simulink model "Planta_FTV_load_balanceada"  (R2020a)
settings: Solver=VariableStepAuto  StartTime=0.0  StopTime=total_sim  MaxStep=1e-4  RelTol=1e-3
values from neighbouring files (symbols this model uses):
  day = 9 + i    [main.m]
  duty_solar = (4*rand())-(3*rand())+90    [main.m]
  gain_time = 0.0001    [main.m]
  L1 = 8.5e-03 + rand()*1e-04    [main.m]
  L2 = 12e-03 + rand()*1e-04    [main.m]
  L3 = 19e-03 + rand()*1e-04    [main.m]
  L4 = 18e-03 + rand()*1e-04    [main.m]
  L5 = 12e-03 + rand()*1e-04    [main.m]
  R = 10    [main.m]
  T1 = 2 *time_hour + rand()*0.5    [main.m]
  T2 = 6 *time_hour + rand()*0.5    [main.m]
  T3 = 11 *time_hour + rand()*0.5    [main.m]
  T4 = 17 * time_hour + rand()*0.5    [main.m]
  T5 = 18    [main.m]
  total_sim = (horas_simular*60*60)*gain_time    (= 0.18)    [main.m]
  ts_save = gain_time *10    (= 0.001)    [main.m]
  ts_send = 0.01    [main.m]
  weekday = 1 +i    [main.m]
libraries: powerlib x45, powerlib_meascontrol x9, simulink x2, instrumentlib x2, eePowerMeasurement x1, powerlib_extras x1, re_lib x1
settings Model: Creator=Daniel Gusnay  LastModifiedBy=bazur
settings DataIOCC: ReturnWorkspaceOutputs=off
settings DebuggingCC: ArithmeticOperatorsInVariantConditions=warning
settings SFSimCC: SimUseLocalCustomCode=off  CustomCodeUndefinedFunction=UseInterfaceOnly
settings RTWCC: RTWUseLocalCustomCode=off

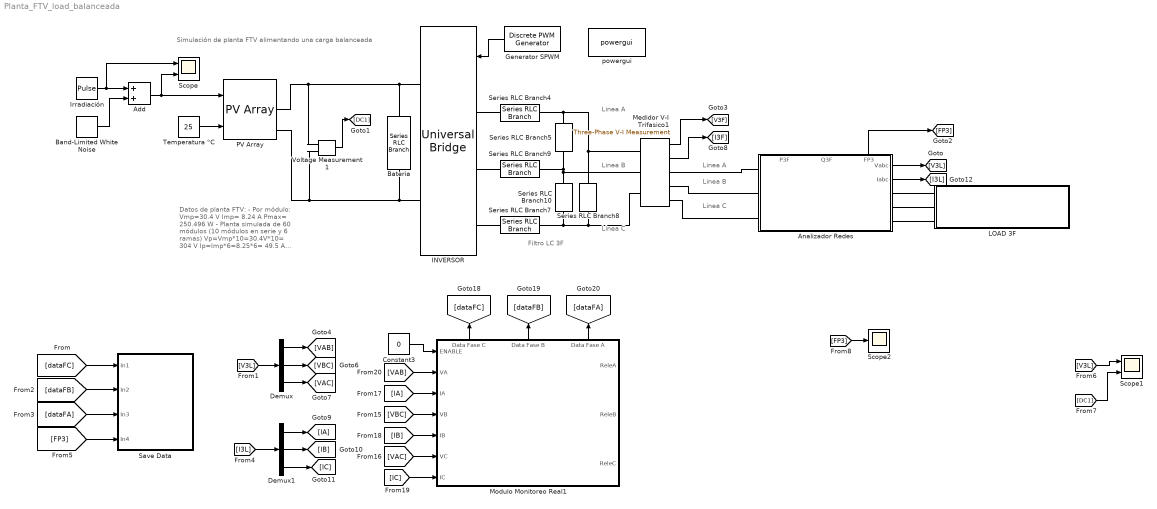
== system Planta_FTV_load_balanceada ==
  note: Simulación de planta FTV alimentando una carga balanceada
  note: Filtro LC 3F
  note: Datos de planta FTV:
      | - Por módulo:
      | Vmp=30.4 V
      | Imp= 8.24 A
      | Pmax= 250.496 W
      | - Planta simulada de 60 módulos
      | (10 módulos en serie y 6 ramas)
      | Vp=Vmp*10=30.4V*10= 304 V
      | Ip=Imp*6=8.25*6= 49.5 A
      | Pp=250.496*60= 15.03 KW
  note: Linea C
  note: Linea A
  note: Linea B
  note: Linea B
  note: Linea C
  note: Linea A
  Add : Sum
  Analizador Redes : Subsystem
      settings: PortSchema="{\"entries\":[{\"content\":{\"sides\":[{\"content\":{\"connectorIds\":[\"LConn1\",\"LConn2\",\"LConn3\"]},\"type\":\"ConnectorPlacement.EquallySpacedRectSide\",\"uuid\":\"8d217d1e-5ed8-457e-9d73-5f3c4b7e42f8\"},{\"content\":{\"connectorIds\":[\"Out1\",\"Out2\",\"RConn1\",\"RConn2\",\"RConn3\"],\"side\":\"RIGHT\"},\"type\":\"ConnectorPlacement.EquallySpacedRectSide\",\"uuid\":\"96ffc5ce-4bc1-4fd3-932f-b78e24123536\"},{\"content\":{\"connectorIds\":[\"Out3\",\"Out4\",\"Out5\"],\"side\":\"TOP\"},\"type\":\"ConnectorPlacement.EquallySpacedRectSide\",\"uuid\":\"fc9d1790-d6c7-48c1-8dca-487e5e9ed0da\"}]},\"type\":\"ConnectorPlacement.EquallySpacedConnector\",\"uuid\":\"142490fa-0bc6-467b-8a94-c7fb7694c71d\"}],\"packageUris\":[\"http://schema.mathworks.com/mf0/Connector/19700101\"],\"version\":\"1.0\"}"
  Band-Limited White Noise : simulink/Sources/Band-Limited White Noise  Cov=[0.1]  Ts=ts_save  seed=speed_solar
  Bateria : powerlib/Elements/Series RLC Branch  LConnTagsString=__new0  RConnTagsString=__new0  BranchType=C  Resistance=1  Inductance=1e-3  SetiL0=off  InitialCurrent=0  Capacitance=0.001  Setx0=on  InitialVoltage=0  Measurements=None
  Constant3 : Constant  Value=0
  Demux : Demux  Outputs=3
  Demux1 : Demux  Outputs=3
  "Generator SPWM " : powerlib_extras/Discrete  Control Blocks/Discrete PWM Generator  GeneratorMode="3-arm  bridge (6 pulses)"  Fc=1080  Ts=5.14e-6  Internal=on  mIndex=0.85  Freq=60  Phase=0
      settings: SourceProductBaseCode=PS
  INVERSOR : powerlib/Power Electronics/Universal Bridge  Arms=3  SnubberResistance=1e5  SnubberCapacitance=inf  Device=IGBT / Diodes  Ron=1e-3  Lon=0  ForwardVoltages="[  0  0  ]"  ForwardVoltage=0  GTOparameters=[ 10e-6 , 20e-6 ]  IGBTparameters=[ 1e-6 , 2e-6 ]  Measurements=None  Measurements_2=None  converterType=Rectifier
  Irradiación : DiscretePulseGenerator  PulseType=Time based  Amplitude=4000  Period=total_sim  PulseWidth=duty_solar
  LOAD 3F : Subsystem
      settings: PortSchema="{\"entries\":[{\"content\":{\"sides\":[{\"content\":{\"connectorIds\":[]},\"type\":\"ConnectorPlacement.EquallySpacedRectSide\",\"uuid\":\"a45682e9-5641-485a-8354-6e8dd6e723a9\"},{\"content\":{\"connectorIds\":[],\"side\":\"RIGHT\"},\"type\":\"ConnectorPlacement.EquallySpacedRectSide\",\"uuid\":\"7c2ca276-e889-4aec-8b9e-0cffbfa5e25f\"},{\"content\":{\"connectorIds\":[\"LConn1\",\"LConn2\",\"LConn3\"],\"side\":\"TOP\"},\"type\":\"ConnectorPlacement.EquallySpacedRectSide\",\"uuid\":\"db21ef6f-2ee7-4f3e-943d-4e32f0d70509\"}]},\"type\":\"ConnectorPlacement.EquallySpacedConnector\",\"uuid\":\"0b995496-a1d7-4479-b2d0-b083c1819622\"}],\"packageUris\":[\"http://schema.mathworks.com/mf0/Connector/19700101\"],\"version\":\"1.0\"}"
  Medidor V-I Trifasico1 : powerlib/Measurements/Three-Phase V-I Measurement  VoltageMeasurement=phase-to-phase  SetLabelV=off  LabelV=Vabc  Vpu=off  VpuLL=off  CurrentMeasurement=yes  SetLabelI=off  LabelI=Iabc  Ipu=off  Pbase=100e6  Vbase=500e3  OutputType=Complex  PhasorSimulation=off  PSBequivalent=0
  Modulo Monitoreo Real1 : Subsystem
      settings: PortSchema="{\"entries\":[{\"content\":{\"sides\":[{\"content\":{\"connectorIds\":[\"In1\",\"In2\",\"In3\",\"In4\",\"In5\",\"In6\",\"In7\"]},\"type\":\"ConnectorPlacement.EquallySpacedRectSide\",\"uuid\":\"f726b031-035b-4703-af3f-a4e51d0dca98\"},{\"content\":{\"connectorIds\":[\"Out1\",\"Out2\",\"Out3\"],\"side\":\"RIGHT\"},\"type\":\"ConnectorPlacement.EquallySpacedRectSide\",\"uuid\":\"d317a734-42d7-4878-a87e-3ae99e4df09f\"},{\"content\":{\"connectorIds\":[\"Out4\",\"Out5\",\"Out6\"],\"side\":\"TOP\"},\"type\":\"ConnectorPlacement.EquallySpacedRectSide\",\"uuid\":\"3f8ce4c0-84cc-4512-a908-abb1f3fc3c08\"},{\"content\":{\"connectorIds\":[],\"side\":\"BOTTOM\"},\"type\":\"ConnectorPlacement.EquallySpacedRectSide\",\"uuid\":\"95f59266-31ff-4071-9e63-6fbc8f4be1bf\"}]},\"type\":\"ConnectorPlacement.EquallySpacedConnector\",\"uuid\":\"51425b5b-918b-4ee3-8f8a-3aaf36556f32\"}],\"packageUris\":[\"http://schema.mathworks.com/mf0/Connector/19700101\"],\"version\":\"1.0\"}"
      mask Display: image('C:\Users\bazur\Desktop\RedNeuronal\RedNeuronalTesis\matlab\pictures\modulo.jpg'); % Use "Edit Image" on toolstrip to change.
  PV Array : re_lib/Solar/PV Array  Npar=6  Nser=10  PlotType=array @ 1000 W/m2 & specified temperatures  S_vec="[ 1000  500  100 ]"  Temp_C_vec="[ 45 25  ]"  ModuleName=Yingli Energy (China) YL250P-29b  PlotWhenSelected=off  Pm=250.496  Ncell=60  Voc=38.4  Isc=8.79  Vm=30.4  Im=8.24  beta_Voc_pc=-0.33701  alpha_Isc_pc=0.0438  beta_Voc=-0.12941  alpha_Isc=0.00385  IL=8.8002  I0=1.2723e-10  nI=0.9985  Rsh=364.6382  Rs=0.42475  RobustModel=off  RobustCellTemperature=25  BAL=off  Tc=1e-6  Tfilter=5e-5
  Save Data : Subsystem
  Scope : Scope  NumInputPorts=2
  Scope1 : Scope  NumInputPorts=2
  Scope2 : Scope
  Series RLC Branch10 : powerlib/Elements/Series RLC Branch  LConnTagsString=__new0  RConnTagsString=__new0  BranchType=C  Resistance=1  Inductance=1e-3  SetiL0=off  InitialCurrent=0  Capacitance=0.001  Setx0=off  InitialVoltage=0  Measurements=None
  Series RLC Branch4 : powerlib/Elements/Series RLC Branch  LConnTagsString=__new0  RConnTagsString=__new0  BranchType=L  Resistance=1  Inductance=0.007  SetiL0=off  InitialCurrent=0  Capacitance=0.006  Setx0=off  InitialVoltage=0  Measurements=None
  Series RLC Branch5 : powerlib/Elements/Series RLC Branch  LConnTagsString=__new0  RConnTagsString=__new0  BranchType=C  Resistance=1  Inductance=1e-3  SetiL0=off  InitialCurrent=0  Capacitance=0.001  Setx0=off  InitialVoltage=0  Measurements=None
  Series RLC Branch7 : powerlib/Elements/Series RLC Branch  LConnTagsString=__new0  RConnTagsString=__new0  BranchType=L  Resistance=1  Inductance=0.007  SetiL0=off  InitialCurrent=0  Capacitance=0.006  Setx0=off  InitialVoltage=0  Measurements=None
  Series RLC Branch8 : powerlib/Elements/Series RLC Branch  LConnTagsString=__new0  RConnTagsString=__new0  BranchType=C  Resistance=1  Inductance=1e-3  SetiL0=off  InitialCurrent=0  Capacitance=0.001  Setx0=off  InitialVoltage=0  Measurements=None
  Series RLC Branch9 : powerlib/Elements/Series RLC Branch  LConnTagsString=__new0  RConnTagsString=__new0  BranchType=L  Resistance=1  Inductance=0.007  SetiL0=off  InitialCurrent=0  Capacitance=0.006  Setx0=off  InitialVoltage=0  Measurements=None
  Temperatura °C : Constant  Value=25
  Voltage Measurement1 : powerlib/Measurements/Voltage Measurement  PhasorSimulation=off  OutputType=Complex  PSBequivalent=0
  powergui : powerlib/powergui  Priority=1  SimulationMode=Continuous  SampleTime=50e-6  frequency=60  Iterations=50  frequencyindice=0  Pbase=100e6  ErrMax=1e-4  UnitsV=kV  UnitsW=MW  buscounter=0  FunctionMessages=off  echomessages=off  EnableUseOfTLC=off  CurrentSourceSwitches=off  DisableSnubberDevices=off  DisableRonSwitches=off  DisableVfSwitches=off  DisplayEquations=off  AutomaticDiscreteSolvers=off  SolverType=Tustin/Backward Euler (TBE)  Interpol=off  ExternalGateDelay=off  methode=off  Ts=100  x0status=blocks  SPID=on  SwTol=0  HookPort=off  NonlinearTolerance=1e-4  nMaxIteration=100  ContinueOnMaxIteration=off  RestoreLinks=warning  ResistiveCurrentMeasurement=off  Frange=[0:2:500]  Ylog=off  Xlog=on  ShowGrid=off  save=off  variable=ZData  structure=0  ZoomFFT=off  StartTime=0.0  cycles=1  DisplayStyle=1  fundamental=60  FreqAxis=off  MaxFrequency=1000  frequencyindicesteady=1  RmsSteady=1  display=off
  wires:
  Temperatura °C/1 -> PV Array/2
  Voltage Measurement1/1 -> [DC1]
  "Generator SPWM "/1 -> INVERSOR/1
  Medidor V-I Trifasico1/1 -> [V3F]
  Medidor V-I Trifasico1/2 -> [I3F]
  [V3L] -> Demux/1
  [I3L] -> Demux1/1
  Demux/1 -> [VAB]
  Demux/2 -> [VBC]
  Demux/3 -> [VAC]
  Demux1/3 -> [IC]
  Demux1/1 -> [IA]
  Demux1/2 -> [IB]
  [IB] -> Modulo Monitoreo Real1/5(IB)
  [IC] -> Modulo Monitoreo Real1/7(IC)
  [VAB] -> Modulo Monitoreo Real1/2(VA)
  Constant3/1 -> Modulo Monitoreo Real1/1(ENABLE)
  [VAC] -> Modulo Monitoreo Real1/6(VC)
  [VBC] -> Modulo Monitoreo Real1/4(VB)
  [IA] -> Modulo Monitoreo Real1/3(IA)
  Modulo Monitoreo Real1/4(Data Fase C) -> [dataFC]
  Modulo Monitoreo Real1/5(Data Fase B) -> [dataFB]
  Modulo Monitoreo Real1/6(Data Fase A) -> [dataFA]
  Analizador Redes/1(Vabc) -> [V3L]
  Analizador Redes/2(Iabc) -> [I3L]
  Analizador Redes/5(FP3) -> [FP3]
  Irradiación/1 -> Scope/1, Add/1
  Band-Limited White Noise/1 -> Add/2
  Add/1 -> Scope/2, PV Array/1
  [V3L] -> Scope1/1
  [DC1] -> Scope1/2
  [dataFC] -> Save Data/1(In1)
  [dataFB] -> Save Data/2(In2)
  [dataFA] -> Save Data/3(In3)
  [FP3] -> Save Data/4(In4)
  [FP3] -> Scope2/1
  connections:
  Bateria/LConn1 -- PV Array/RConn1 -- Voltage Measurement1/LConn1 -- INVERSOR/RConn1
  Series RLC Branch4/LConn1 -- Series RLC Branch5/LConn1 -- Medidor V-I Trifasico1/LConn1 -- Series RLC Branch8/LConn1
  Bateria/RConn1 -- PV Array/RConn2 -- Voltage Measurement1/LConn2 -- INVERSOR/RConn2
  Series RLC Branch7/RConn1 -- INVERSOR/LConn3
  Series RLC Branch9/RConn1 -- INVERSOR/LConn2
  Series RLC Branch4/RConn1 -- INVERSOR/LConn1
  Series RLC Branch10/LConn1 -- Series RLC Branch5/RConn1 -- Series RLC Branch9/LConn1 -- Medidor V-I Trifasico1/LConn2
  Series RLC Branch8/RConn1 -- Series RLC Branch7/LConn1 -- Series RLC Branch10/RConn1 -- Medidor V-I Trifasico1/LConn3
  Medidor V-I Trifasico1/RConn2 -- Analizador Redes/LConn2
  Medidor V-I Trifasico1/RConn3 -- Analizador Redes/LConn3
  Medidor V-I Trifasico1/RConn1 -- Analizador Redes/LConn1
  Analizador Redes/RConn1 -- LOAD 3F/LConn1
  Analizador Redes/RConn2 -- LOAD 3F/LConn2
  Analizador Redes/RConn3 -- LOAD 3F/LConn3

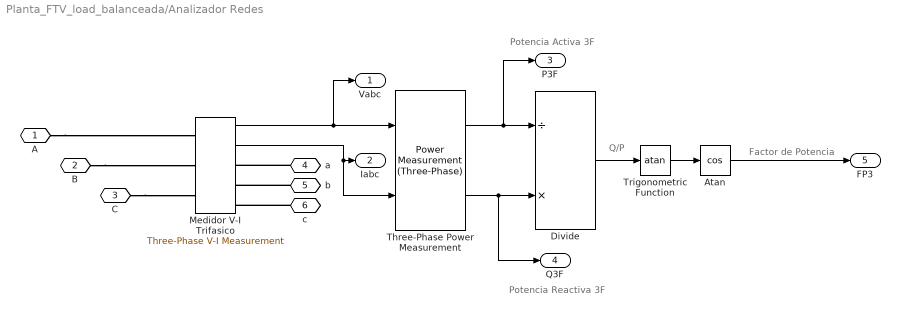
== system Planta_FTV_load_balanceada/Analizador Redes ==
  note: Q/P
  note: Potencia Activa 3F
  note: Potencia Reactiva 3F
  note: Factor de Potencia
  Atan : Trigonometry  Operator=cos
  Divide : Product  Inputs=/*
  Medidor V-I Trifasico : powerlib/Measurements/Three-Phase V-I Measurement  VoltageMeasurement=phase-to-phase  SetLabelV=off  LabelV=Vabc  Vpu=off  VpuLL=off  CurrentMeasurement=yes  SetLabelI=off  LabelI=Iabc  Ipu=off  Pbase=100e6  Vbase=500e3  OutputType=Complex  PhasorSimulation=off  PSBequivalent=0
  Three-Phase Power Measurement : eePowerMeasurement/Power Measurement (Three-Phase)  LabelModeActiveChoice=Continuous  F=60  K=[1]  Seq=Positive  Ts=0
      settings: SourceProductBaseCode=PS
  Trigonometric Function : Trigonometry  Operator=atan
  A : PMIOPort  Side=Left
  B : PMIOPort  Port=2  Side=Left
  C : PMIOPort  Port=3  Side=Left
  a : PMIOPort  Port=4  Side=Right
  b : PMIOPort  Port=5  Side=Right
  c : PMIOPort  Port=6  Side=Right
  Vabc : Outport
  Iabc : Outport  Port=2
  P3F : Outport  Port=3
  Q3F : Outport  Port=4
  FP3 : Outport  Port=5
  wires:
  Medidor V-I Trifasico/2 -> Iabc/1, Three-Phase Power Measurement/2
  Divide/1 -> Trigonometric Function/1
  Medidor V-I Trifasico/1 -> Vabc/1, Three-Phase Power Measurement/1
  Three-Phase Power Measurement/1 -> P3F/1, Divide/1
  Three-Phase Power Measurement/2 -> Q3F/1, Divide/2
  Trigonometric Function/1 -> Atan/1
  Atan/1 -> FP3/1
  connections:
  B/RConn1 -- Medidor V-I Trifasico/LConn2
  c/RConn1 -- Medidor V-I Trifasico/RConn3
  b/RConn1 -- Medidor V-I Trifasico/RConn2
  C/RConn1 -- Medidor V-I Trifasico/LConn3
  A/RConn1 -- Medidor V-I Trifasico/LConn1
  a/RConn1 -- Medidor V-I Trifasico/RConn1

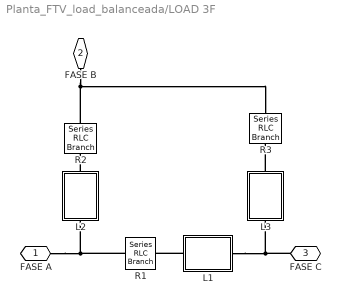
== system Planta_FTV_load_balanceada/LOAD 3F ==
  L1 : Subsystem
      mask Display: image('C:\Users\Daniel Gusnay\Downloads\Inductor_variable.png');
  L2 : Subsystem
      mask Display: image('C:\Users\Daniel Gusnay\Downloads\Inductor_variable.png');
  L3 : Subsystem
      mask Display: image('C:\Users\Daniel Gusnay\Downloads\Inductor_variable.png');
  R1 : powerlib/Elements/Series RLC Branch  LConnTagsString=__new0  RConnTagsString=__new0  BranchType=R  Resistance=R  Inductance=40e-3  SetiL0=on  InitialCurrent=0  Capacitance=0.006  Setx0=off  InitialVoltage=0  Measurements=None
  R2 : powerlib/Elements/Series RLC Branch  LConnTagsString=__new0  RConnTagsString=__new0  BranchType=R  Resistance=R  Inductance=40e-3  SetiL0=on  InitialCurrent=0  Capacitance=0.006  Setx0=off  InitialVoltage=0  Measurements=None
  R3 : powerlib/Elements/Series RLC Branch  LConnTagsString=__new0  RConnTagsString=__new0  BranchType=R  Resistance=R  Inductance=40e-3  SetiL0=on  InitialCurrent=0  Capacitance=0.006  Setx0=off  InitialVoltage=0  Measurements=None
  FASE A : PMIOPort  Side=Left
  FASE B : PMIOPort  Port=2  Side=Left
  FASE C : PMIOPort  Port=3  Side=Left
  connections:
  L3/RConn1 -- R3/LConn1
  L1/LConn1 -- R1/RConn1
  L2/LConn1 -- R2/RConn1
  R1/LConn1 -- FASE A/RConn1 -- L2/RConn1
  L1/RConn1 -- FASE C/RConn1 -- L3/LConn1
  R2/LConn1 -- FASE B/RConn1 -- R3/RConn1

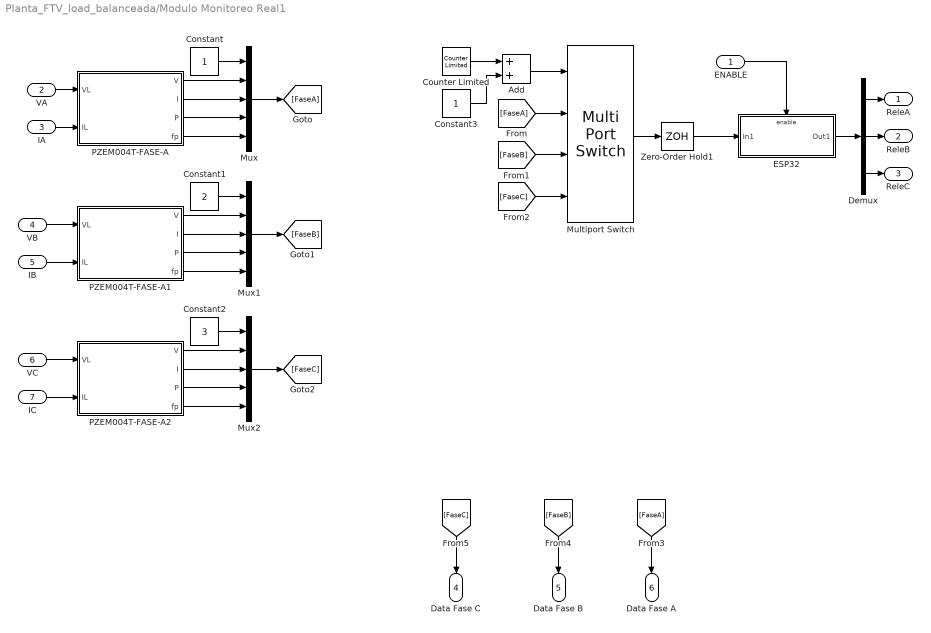
== system Planta_FTV_load_balanceada/Modulo Monitoreo Real1 ==
  ENABLE : Inport
  VA : Inport  Port=2
  IA : Inport  Port=3
  VB : Inport  Port=4
  IB : Inport  Port=5
  VC : Inport  Port=6
  IC : Inport  Port=7
  Add : Sum
  Constant : Constant
  Constant1 : Constant  Value=2
  Constant2 : Constant  Value=3
  Constant3 : Constant
  Counter Limited : simulink/Sources/Counter Limited  uplimit=2  tsamp=ts_send
  Demux : Demux  Outputs=3
  ESP32 : Subsystem  TreatAsAtomicUnit=on
  Multiport Switch : MultiPortSwitch
  Mux : Mux  Inputs=5
  Mux1 : Mux  Inputs=5
  Mux2 : Mux  Inputs=5
  PZEM004T-FASE-A : Subsystem
      mask Display: image('C:\Users\bazur\Desktop\RedNeuronal\RedNeuronalTesis\matlab\pictures\PZEM-004-module.jpg'); % Use "Edit Image" on toolstrip to change.
  PZEM004T-FASE-A1 : Subsystem
      mask Display: image('C:\Users\bazur\Desktop\RedNeuronal\RedNeuronalTesis\matlab\pictures\PZEM-004-module.jpg'); % Use "Edit Image" on toolstrip to change.
  PZEM004T-FASE-A2 : Subsystem
      mask Display: image('C:\Users\bazur\Desktop\RedNeuronal\RedNeuronalTesis\matlab\pictures\PZEM-004-module.jpg'); % Use "Edit Image" on toolstrip to change.
  Zero-Order Hold1 : ZeroOrderHold  SampleTime=ts_send
  ReleA : Outport
  ReleB : Outport  Port=2
  ReleC : Outport  Port=3
  Data Fase C : Outport  Port=4
  Data Fase B : Outport  Port=5
  Data Fase A : Outport  Port=6
  wires:
  VA/1 -> PZEM004T-FASE-A/1(VL)
  IA/1 -> PZEM004T-FASE-A/2(IL)
  IB/1 -> PZEM004T-FASE-A1/2(IL)
  VB/1 -> PZEM004T-FASE-A1/1(VL)
  PZEM004T-FASE-A/1(V) -> Mux/2
  PZEM004T-FASE-A/2(I) -> Mux/3
  PZEM004T-FASE-A/3(P) -> Mux/4
  PZEM004T-FASE-A/4(fp) -> Mux/5
  Constant/1 -> Mux/1
  Mux/1 -> [FaseA]
  [FaseA] -> Multiport Switch/2
  Constant1/1 -> Mux1/1
  Mux1/1 -> [FaseB]
  PZEM004T-FASE-A1/2(I) -> Mux1/3
  PZEM004T-FASE-A1/4(fp) -> Mux1/5
  PZEM004T-FASE-A1/1(V) -> Mux1/2
  PZEM004T-FASE-A1/3(P) -> Mux1/4
  Constant2/1 -> Mux2/1
  VC/1 -> PZEM004T-FASE-A2/1(VL)
  PZEM004T-FASE-A2/3(P) -> Mux2/4
  IC/1 -> PZEM004T-FASE-A2/2(IL)
  PZEM004T-FASE-A2/4(fp) -> Mux2/5
  PZEM004T-FASE-A2/1(V) -> Mux2/2
  Mux2/1 -> [FaseC]
  PZEM004T-FASE-A2/2(I) -> Mux2/3
  [FaseB] -> Multiport Switch/3
  [FaseC] -> Multiport Switch/4
  Counter Limited/1 -> Add/1
  Add/1 -> Multiport Switch/1
  Constant3/1 -> Add/2
  Multiport Switch/1 -> Zero-Order Hold1/1
  [FaseB] -> Data Fase B/1
  [FaseC] -> Data Fase C/1
  Demux/2 -> ReleB/1
  Demux/1 -> ReleA/1
  Demux/3 -> ReleC/1
  [FaseA] -> Data Fase A/1
  Zero-Order Hold1/1 -> ESP32/1(In1)
  ESP32/1(Out1) -> Demux/1
  ENABLE/1 -> ESP32/Enable

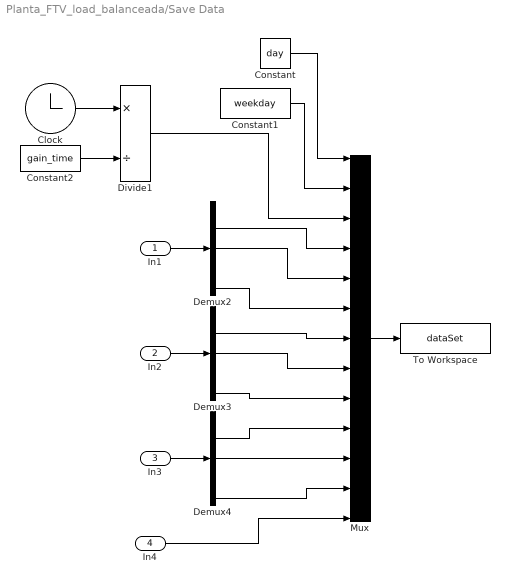
== system Planta_FTV_load_balanceada/Save Data ==
  In1 : Inport
  In2 : Inport  Port=2
  In3 : Inport  Port=3
  In4 : Inport  Port=4
  Clock : Clock
  Constant : Constant  Value=day
  Constant1 : Constant  Value=weekday
  Constant2 : Constant  Value=gain_time
  Demux2 : Demux  Outputs=5
  Demux3 : Demux  Outputs=5
  Demux4 : Demux  Outputs=5
  Divide1 : Product  Inputs=*/
  Mux : Mux  Inputs=13
  To Workspace : ToWorkspace  VariableName=dataSet  SampleTime=ts_save
  wires:
  Demux3/2 -> Mux/7
  Demux3/5 -> Mux/9
  Demux4/2 -> Mux/10
  Mux/1 -> To Workspace/1
  Demux2/3 -> Mux/5
  Demux2/2 -> Mux/4
  Demux3/3 -> Mux/8
  In3/1 -> Demux4/1
  Demux4/5 -> Mux/12
  Demux4/3 -> Mux/11
  Constant2/1 -> Divide1/2
  Clock/1 -> Divide1/1
  Constant1/1 -> Mux/2
  Constant/1 -> Mux/1
  Demux2/5 -> Mux/6
  In1/1 -> Demux2/1
  Divide1/1 -> Mux/3
  In4/1 -> Mux/13
  In2/1 -> Demux3/1

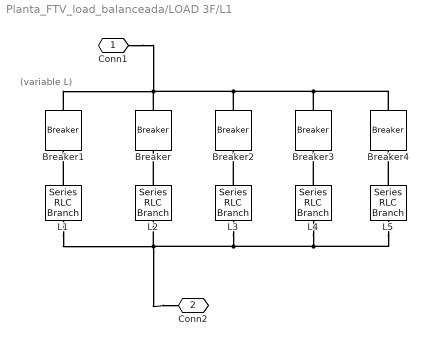
== system Planta_FTV_load_balanceada/LOAD 3F/L1 ==
  note: (variable L)
  Breaker : powerlib/Elements/Breaker  InitialState=0  SwitchingTimes=[T1 T2]  External=off  BreakerResistance=0.01  SnubberResistance=1e6  SnubberCapacitance=inf  Measurements=None  MoreParameters=on  NoBreakLoop=off
  Breaker1 : powerlib/Elements/Breaker  InitialState=0  SwitchingTimes="[0  T1]"  External=off  BreakerResistance=0.01  SnubberResistance=1e6  SnubberCapacitance=inf  Measurements=None  MoreParameters=on  NoBreakLoop=off
  Breaker2 : powerlib/Elements/Breaker  InitialState=0  SwitchingTimes="[T2  T3]"  External=off  BreakerResistance=0.01  SnubberResistance=1e6  SnubberCapacitance=inf  Measurements=None  MoreParameters=on  NoBreakLoop=off
  Breaker3 : powerlib/Elements/Breaker  InitialState=0  SwitchingTimes="[T3  T4]"  External=off  BreakerResistance=0.01  SnubberResistance=1e6  SnubberCapacitance=inf  Measurements=None  MoreParameters=on  NoBreakLoop=off
  Breaker4 : powerlib/Elements/Breaker  InitialState=0  SwitchingTimes="[T4  T5]"  External=off  BreakerResistance=0.01  SnubberResistance=1e6  SnubberCapacitance=inf  Measurements=None  MoreParameters=on  NoBreakLoop=off
  L1 : powerlib/Elements/Series RLC Branch  LConnTagsString=__new0  RConnTagsString=__new0  BranchType=L  Resistance=R  Inductance=L1  SetiL0=off  InitialCurrent=0  Capacitance=0.006  Setx0=off  InitialVoltage=0  Measurements=None
  L2 : powerlib/Elements/Series RLC Branch  LConnTagsString=__new0  RConnTagsString=__new0  BranchType=L  Resistance=R  Inductance=L2  SetiL0=off  InitialCurrent=0  Capacitance=0.006  Setx0=off  InitialVoltage=0  Measurements=None
  L3 : powerlib/Elements/Series RLC Branch  LConnTagsString=__new0  RConnTagsString=__new0  BranchType=L  Resistance=R  Inductance=L3  SetiL0=off  InitialCurrent=0  Capacitance=0.006  Setx0=off  InitialVoltage=0  Measurements=None
  L4 : powerlib/Elements/Series RLC Branch  LConnTagsString=__new0  RConnTagsString=__new0  BranchType=L  Resistance=R  Inductance=L4  SetiL0=off  InitialCurrent=0  Capacitance=0.006  Setx0=off  InitialVoltage=0  Measurements=None
  L5 : powerlib/Elements/Series RLC Branch  LConnTagsString=__new0  RConnTagsString=__new0  BranchType=L  Resistance=R  Inductance=L5  SetiL0=off  InitialCurrent=0  Capacitance=0.006  Setx0=off  InitialVoltage=0  Measurements=None
  Conn1 : PMIOPort  Side=Left
  Conn2 : PMIOPort  Port=2  Side=Right
  connections:
  Conn2/RConn1 -- L5/RConn1 -- L4/RConn1 -- L3/RConn1 -- L2/RConn1 -- L1/RConn1
  L3/LConn1 -- Breaker2/LConn1
  L1/LConn1 -- Breaker1/LConn1
  L2/LConn1 -- Breaker/LConn1
  Conn1/RConn1 -- Breaker4/RConn1 -- Breaker3/RConn1 -- Breaker2/RConn1 -- Breaker/RConn1 -- Breaker1/RConn1
  L4/LConn1 -- Breaker3/LConn1
  L5/LConn1 -- Breaker4/LConn1

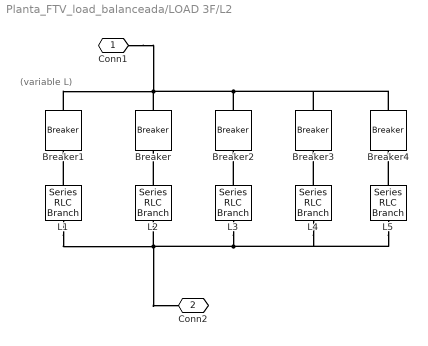
== system Planta_FTV_load_balanceada/LOAD 3F/L2 ==
  note: (variable L)
  Breaker : powerlib/Elements/Breaker  InitialState=0  SwitchingTimes=[T1 T2]  External=off  BreakerResistance=0.01  SnubberResistance=1e6  SnubberCapacitance=inf  Measurements=None  MoreParameters=on  NoBreakLoop=off
  Breaker1 : powerlib/Elements/Breaker  InitialState=0  SwitchingTimes="[0  T1]"  External=off  BreakerResistance=0.01  SnubberResistance=1e6  SnubberCapacitance=inf  Measurements=None  MoreParameters=on  NoBreakLoop=off
  Breaker2 : powerlib/Elements/Breaker  InitialState=0  SwitchingTimes="[T2  T3]"  External=off  BreakerResistance=0.01  SnubberResistance=1e6  SnubberCapacitance=inf  Measurements=None  MoreParameters=on  NoBreakLoop=off
  Breaker3 : powerlib/Elements/Breaker  InitialState=0  SwitchingTimes="[T3  T4]"  External=off  BreakerResistance=0.01  SnubberResistance=1e6  SnubberCapacitance=inf  Measurements=None  MoreParameters=on  NoBreakLoop=off
  Breaker4 : powerlib/Elements/Breaker  InitialState=0  SwitchingTimes="[T4  T5]"  External=off  BreakerResistance=0.01  SnubberResistance=1e6  SnubberCapacitance=inf  Measurements=None  MoreParameters=on  NoBreakLoop=off
  L1 : powerlib/Elements/Series RLC Branch  LConnTagsString=__new0  RConnTagsString=__new0  BranchType=L  Resistance=R  Inductance=L1  SetiL0=off  InitialCurrent=0  Capacitance=0.006  Setx0=off  InitialVoltage=0  Measurements=None
  L2 : powerlib/Elements/Series RLC Branch  LConnTagsString=__new0  RConnTagsString=__new0  BranchType=L  Resistance=R  Inductance=L2  SetiL0=off  InitialCurrent=0  Capacitance=0.006  Setx0=off  InitialVoltage=0  Measurements=None
  L3 : powerlib/Elements/Series RLC Branch  LConnTagsString=__new0  RConnTagsString=__new0  BranchType=L  Resistance=R  Inductance=L3  SetiL0=off  InitialCurrent=0  Capacitance=0.006  Setx0=off  InitialVoltage=0  Measurements=None
  L4 : powerlib/Elements/Series RLC Branch  LConnTagsString=__new0  RConnTagsString=__new0  BranchType=L  Resistance=R  Inductance=L4  SetiL0=off  InitialCurrent=0  Capacitance=0.006  Setx0=off  InitialVoltage=0  Measurements=None
  L5 : powerlib/Elements/Series RLC Branch  LConnTagsString=__new0  RConnTagsString=__new0  BranchType=L  Resistance=R  Inductance=L5  SetiL0=off  InitialCurrent=0  Capacitance=0.006  Setx0=off  InitialVoltage=0  Measurements=None
  Conn1 : PMIOPort  Side=Left
  Conn2 : PMIOPort  Port=2  Side=Right
  connections:
  L5/LConn1 -- Breaker4/LConn1
  L4/LConn1 -- Breaker3/LConn1
  Breaker1/RConn1 -- Breaker/RConn1 -- Breaker2/RConn1 -- Breaker3/RConn1 -- Breaker4/RConn1 -- Conn1/RConn1
  L2/LConn1 -- Breaker/LConn1
  L1/LConn1 -- Breaker1/LConn1
  L3/LConn1 -- Breaker2/LConn1
  L1/RConn1 -- L2/RConn1 -- L3/RConn1 -- L4/RConn1 -- L5/RConn1 -- Conn2/RConn1

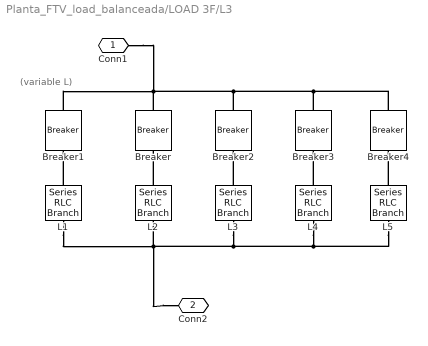
== system Planta_FTV_load_balanceada/LOAD 3F/L3 ==
  note: (variable L)
  Breaker : powerlib/Elements/Breaker  InitialState=0  SwitchingTimes=[T1 T2]  External=off  BreakerResistance=0.01  SnubberResistance=1e6  SnubberCapacitance=inf  Measurements=None  MoreParameters=on  NoBreakLoop=off
  Breaker1 : powerlib/Elements/Breaker  InitialState=0  SwitchingTimes="[0  T1]"  External=off  BreakerResistance=0.01  SnubberResistance=1e6  SnubberCapacitance=inf  Measurements=None  MoreParameters=on  NoBreakLoop=off
  Breaker2 : powerlib/Elements/Breaker  InitialState=0  SwitchingTimes="[T2  T3]"  External=off  BreakerResistance=0.01  SnubberResistance=1e6  SnubberCapacitance=inf  Measurements=None  MoreParameters=on  NoBreakLoop=off
  Breaker3 : powerlib/Elements/Breaker  InitialState=0  SwitchingTimes="[T3  T4]"  External=off  BreakerResistance=0.01  SnubberResistance=1e6  SnubberCapacitance=inf  Measurements=None  MoreParameters=on  NoBreakLoop=off
  Breaker4 : powerlib/Elements/Breaker  InitialState=0  SwitchingTimes="[T4  T5]"  External=off  BreakerResistance=0.01  SnubberResistance=1e6  SnubberCapacitance=inf  Measurements=None  MoreParameters=on  NoBreakLoop=off
  L1 : powerlib/Elements/Series RLC Branch  LConnTagsString=__new0  RConnTagsString=__new0  BranchType=L  Resistance=R  Inductance=L1  SetiL0=off  InitialCurrent=0  Capacitance=0.006  Setx0=off  InitialVoltage=0  Measurements=None
  L2 : powerlib/Elements/Series RLC Branch  LConnTagsString=__new0  RConnTagsString=__new0  BranchType=L  Resistance=R  Inductance=L2  SetiL0=off  InitialCurrent=0  Capacitance=0.006  Setx0=off  InitialVoltage=0  Measurements=None
  L3 : powerlib/Elements/Series RLC Branch  LConnTagsString=__new0  RConnTagsString=__new0  BranchType=L  Resistance=R  Inductance=L3  SetiL0=off  InitialCurrent=0  Capacitance=0.006  Setx0=off  InitialVoltage=0  Measurements=None
  L4 : powerlib/Elements/Series RLC Branch  LConnTagsString=__new0  RConnTagsString=__new0  BranchType=L  Resistance=R  Inductance=L4  SetiL0=off  InitialCurrent=0  Capacitance=0.006  Setx0=off  InitialVoltage=0  Measurements=None
  L5 : powerlib/Elements/Series RLC Branch  LConnTagsString=__new0  RConnTagsString=__new0  BranchType=L  Resistance=R  Inductance=L5  SetiL0=off  InitialCurrent=0  Capacitance=0.006  Setx0=off  InitialVoltage=0  Measurements=None
  Conn1 : PMIOPort  Side=Left
  Conn2 : PMIOPort  Port=2  Side=Right
  connections:
  Conn2/RConn1 -- L5/RConn1 -- L4/RConn1 -- L3/RConn1 -- L2/RConn1 -- L1/RConn1
  L3/LConn1 -- Breaker2/LConn1
  L1/LConn1 -- Breaker1/LConn1
  L2/LConn1 -- Breaker/LConn1
  Conn1/RConn1 -- Breaker4/RConn1 -- Breaker3/RConn1 -- Breaker2/RConn1 -- Breaker/RConn1 -- Breaker1/RConn1
  L4/LConn1 -- Breaker3/LConn1
  L5/LConn1 -- Breaker4/LConn1

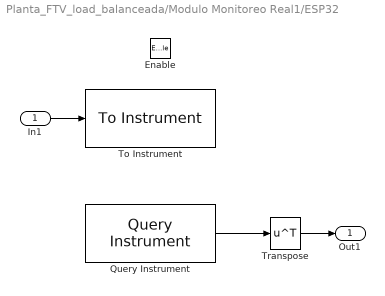
== system Planta_FTV_load_balanceada/Modulo Monitoreo Real1/ESP32 ==
  In1 : Inport
  Enable : EnablePort
  Query Instrument : instrumentlib/Query Instrument  sampleTime=ts_read  isWorkspaceObject=off  timeout=10  inputBufferSize=1012  protocol=Serial  serialPort=COM1  baudRate=115200  gpibVendor=Keysight Technologies  boardIndex=0  primaryAddress=1  secondaryAddress=0  visaVendor=Keysight  visaSerialPort=0  chassisIndex=0  logicalAddress=0  tcpRemoteHost='127.0.0.1'  tcpRemotePort=4500  udpRemoteHost='127.0.0.1'  udpRemotePort=9090  visaTCPBoardIndex=0  visaTCPRemoteHost='127.0.0.1'  usbBoardIndex=0  usbManufID=0  usbModelCode=0  usbSerialNumber=0  initAction=None  initCommand='DATA:SOURCE CH1'  initFunction=get  queryCommand='rele\n'  responseFormat=ASCII  asciiFormatting=ASCII_read  precision=8-bit integer  byteOrder=Little endian  valuesToRead=1  removeBytes=off  afterOutputAction=Repeat query for new data  enableFrames=on  frameSize=3
      settings: SourceProductBaseCode=IC
  To Instrument : instrumentlib/To Instrument  sampleTime=ts_send  isWorkspaceObject=off  timeout=10  inputBufferSize=725000  protocol=Serial  serialPort=COM1  baudRate=115200  gpibVendor=ICS Electronics  boardIndex=0  primaryAddress=1  secondaryAddress=0  visaVendor=Keysight  visaSerialPort=0  chassisIndex=0  logicalAddress=0  tcpRemoteHost='127.0.0.1'  tcpRemotePort=4500  udpRemoteHost='127.0.0.1'  udpRemotePort=9090  visaTCPBoardIndex=0  visaTCPRemoteHost='127.0.0.1'  usbBoardIndex=0  usbManufID=0  usbModelCode=0  usbSerialNumber=0  initAction=None  initCommand='DATA:SOURCE CH1'  initFunction=get  command=''  sendFormat=ASCII  asciiFormatting=ASCII_send  precision=8-bit integer  byteOrder=Little endian
      settings: SourceProductBaseCode=IC
  Transpose : Math  Operator=transpose  SaturateOnIntegerOverflow=on
  Out1 : Outport
  wires:
  Query Instrument/1 -> Transpose/1
  In1/1 -> To Instrument/1
  Transpose/1 -> Out1/1

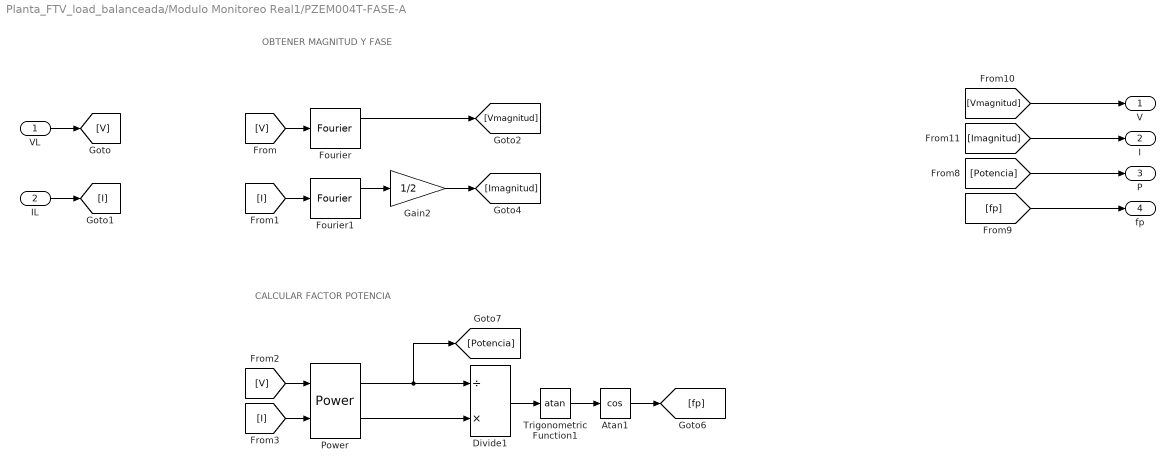
== system Planta_FTV_load_balanceada/Modulo Monitoreo Real1/PZEM004T-FASE-A ==
  note: OBTENER MAGNITUD Y FASE
  note: CALCULAR FACTOR POTENCIA
  VL : Inport
  IL : Inport  Port=2
  Atan1 : Trigonometry  Operator=cos
  Divide1 : Product  Inputs=/*
  Fourier : powerlib_meascontrol/Measurements/Fourier  Freq=60  n=1  InInit=[0, 0]  Ts=0
  Fourier1 : powerlib_meascontrol/Measurements/Fourier  Freq=60  n=1  InInit=[0, 0]  Ts=0
  Gain2 : Gain  Gain=1/2  SaturateOnIntegerOverflow=on  OutDataTypeStr=Inherit: Same as input  ParamDataTypeStr=Inherit: Same as input
  Power : powerlib_meascontrol/Measurements/Power  Freq=60  Vinit=[1, 0]  Iinit=[1, 0]  Ts=0
  Trigonometric Function1 : Trigonometry  Operator=atan
  V : Outport
  I : Outport  Port=2
  P : Outport  Port=3
  fp : Outport  Port=4
  wires:
  VL/1 -> [V]
  [V] -> Fourier/1
  IL/1 -> [I]
  [I] -> Fourier1/1
  [Vmagnitud] -> V/1
  [Imagnitud] -> I/1
  [fp] -> fp/1
  [Potencia] -> P/1
  Divide1/1 -> Trigonometric Function1/1
  Power/2 -> Divide1/2
  Power/1 -> [Potencia], Divide1/1
  Trigonometric Function1/1 -> Atan1/1
  [V] -> Power/1
  [I] -> Power/2
  Atan1/1 -> [fp]
  Fourier/1 -> [Vmagnitud]
  Gain2/1 -> [Imagnitud]
  Fourier1/1 -> Gain2/1

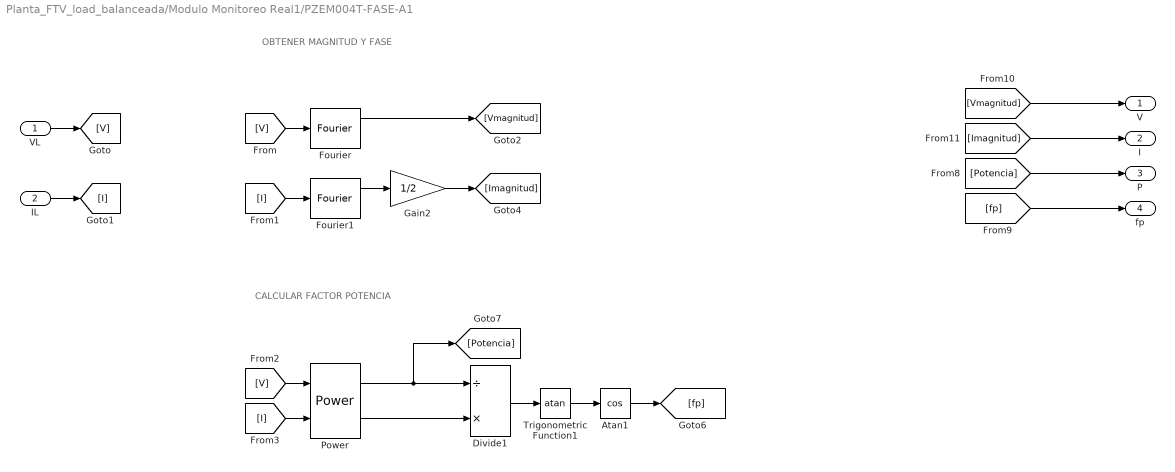
== system Planta_FTV_load_balanceada/Modulo Monitoreo Real1/PZEM004T-FASE-A1 ==
  note: OBTENER MAGNITUD Y FASE
  note: CALCULAR FACTOR POTENCIA
  VL : Inport
  IL : Inport  Port=2
  Atan1 : Trigonometry  Operator=cos
  Divide1 : Product  Inputs=/*
  Fourier : powerlib_meascontrol/Measurements/Fourier  Freq=60  n=1  InInit=[0, 0]  Ts=0
  Fourier1 : powerlib_meascontrol/Measurements/Fourier  Freq=60  n=1  InInit=[0, 0]  Ts=0
  Gain2 : Gain  Gain=1/2  SaturateOnIntegerOverflow=on  OutDataTypeStr=Inherit: Same as input  ParamDataTypeStr=Inherit: Same as input
  Power : powerlib_meascontrol/Measurements/Power  Freq=60  Vinit=[1, 0]  Iinit=[1, 0]  Ts=0
  Trigonometric Function1 : Trigonometry  Operator=atan
  V : Outport
  I : Outport  Port=2
  P : Outport  Port=3
  fp : Outport  Port=4
  wires:
  VL/1 -> [V]
  [V] -> Fourier/1
  IL/1 -> [I]
  [I] -> Fourier1/1
  [Vmagnitud] -> V/1
  [Imagnitud] -> I/1
  [fp] -> fp/1
  [Potencia] -> P/1
  Divide1/1 -> Trigonometric Function1/1
  Power/2 -> Divide1/2
  Power/1 -> [Potencia], Divide1/1
  Trigonometric Function1/1 -> Atan1/1
  [V] -> Power/1
  [I] -> Power/2
  Atan1/1 -> [fp]
  Fourier/1 -> [Vmagnitud]
  Gain2/1 -> [Imagnitud]
  Fourier1/1 -> Gain2/1

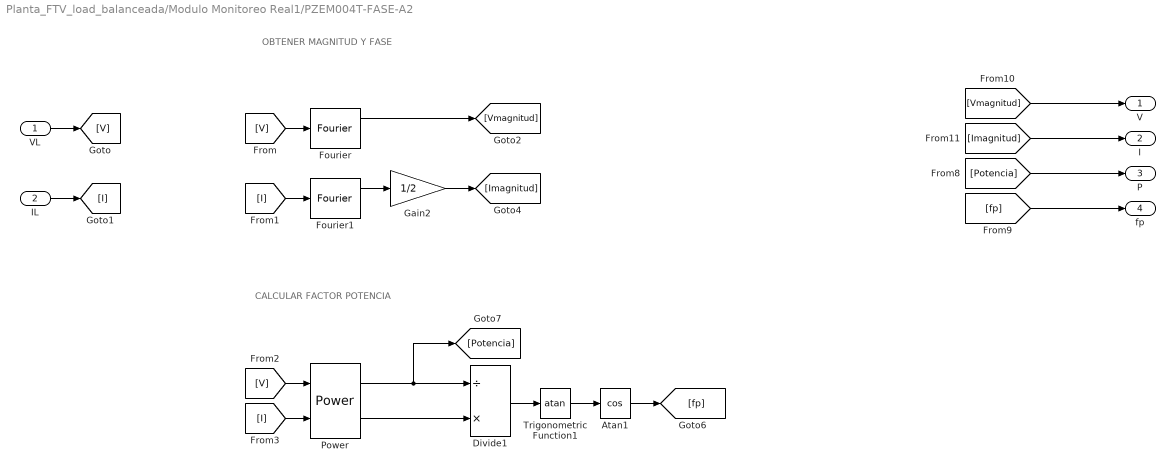
== system Planta_FTV_load_balanceada/Modulo Monitoreo Real1/PZEM004T-FASE-A2 ==
  note: OBTENER MAGNITUD Y FASE
  note: CALCULAR FACTOR POTENCIA
  VL : Inport
  IL : Inport  Port=2
  Atan1 : Trigonometry  Operator=cos
  Divide1 : Product  Inputs=/*
  Fourier : powerlib_meascontrol/Measurements/Fourier  Freq=60  n=1  InInit=[0, 0]  Ts=0
  Fourier1 : powerlib_meascontrol/Measurements/Fourier  Freq=60  n=1  InInit=[0, 0]  Ts=0
  Gain2 : Gain  Gain=1/2  SaturateOnIntegerOverflow=on  OutDataTypeStr=Inherit: Same as input  ParamDataTypeStr=Inherit: Same as input
  Power : powerlib_meascontrol/Measurements/Power  Freq=60  Vinit=[1, 0]  Iinit=[1, 0]  Ts=0
  Trigonometric Function1 : Trigonometry  Operator=atan
  V : Outport
  I : Outport  Port=2
  P : Outport  Port=3
  fp : Outport  Port=4
  wires:
  VL/1 -> [V]
  [V] -> Fourier/1
  IL/1 -> [I]
  [I] -> Fourier1/1
  [Vmagnitud] -> V/1
  [Imagnitud] -> I/1
  [fp] -> fp/1
  [Potencia] -> P/1
  Divide1/1 -> Trigonometric Function1/1
  Power/2 -> Divide1/2
  Power/1 -> [Potencia], Divide1/1
  Trigonometric Function1/1 -> Atan1/1
  [V] -> Power/1
  [I] -> Power/2
  Atan1/1 -> [fp]
  Fourier/1 -> [Vmagnitud]
  Gain2/1 -> [Imagnitud]
  Fourier1/1 -> Gain2/1
